simulink model "PSPCtl_Co"  (R2016b)
settings: configuration reference "CodeGenConfigSet" (kept outside this file)
libraries: CXLib x1
settings Model: Creator=liutao  LastModifiedBy=liutao
settings ConfigSetRef: SourceLocation=Base Workspace

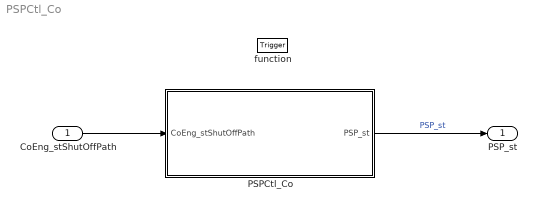
== system PSPCtl_Co ==
  CoEng_stShutOffPath : Inport  Description=Active shut-off paths resulting from active reversible,irreversible and afterrun shut-off paths  OutMin=0  OutMax=65535  OutDataTypeStr=State_uint16
  function : TriggerPort  TriggerType=function-call  VariantControl=Variant
  PSPCtl_Co : Subsystem
  PSP_st : Outport  Description=source for activating the pre-supply pump (1=on/0-=off)  OutMin=0  OutMax=1  OutDataTypeStr=boolean
  wires:
  CoEng_stShutOffPath/1 -> PSPCtl_Co/1(CoEng_stShutOffPath)
  PSPCtl_Co/1(PSP_st) -> PSP_st/1  "PSP_st"

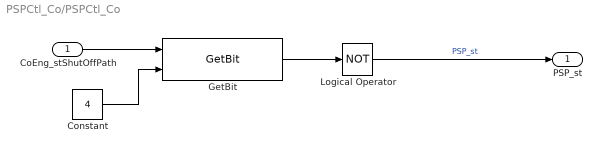
== system PSPCtl_Co/PSPCtl_Co ==
  CoEng_stShutOffPath : Inport  Description=Active shut-off paths resulting from active reversible,irreversible and afterrun shut-off paths  OutMin=0  OutMax=65535  OutDataTypeStr=State_uint16
  Constant : Constant  Value=4  OutDataTypeStr=uint8
  GetBit : CXLib/GetBit  dataTypeString=uint16  dataLength=0
      settings: AttributesFormatString=Get bit from %<dataTypeString>
  Logical Operator : Logic  Operator=NOT  AllPortsSameDT=off  OutDataTypeStr=boolean
  PSP_st : Outport  Description=source for activating the pre-supply pump (1=on/0-=off)  OutMin=0  OutMax=1  OutDataTypeStr=boolean
  wires:
  CoEng_stShutOffPath/1 -> GetBit/1
  Constant/1 -> GetBit/2
  Logical Operator/1 -> PSP_st/1  "PSP_st"
  GetBit/1 -> Logical Operator/1
